simulink model "PowertrainModel"  (R2026b)
settings: Solver=VariableStepAuto
undefined symbols (not defined in the file): Powertrain
settings Model: DataDictionary=VehicleData.sldd  Creator=Xu Dingyi  LastModifiedBy=29358

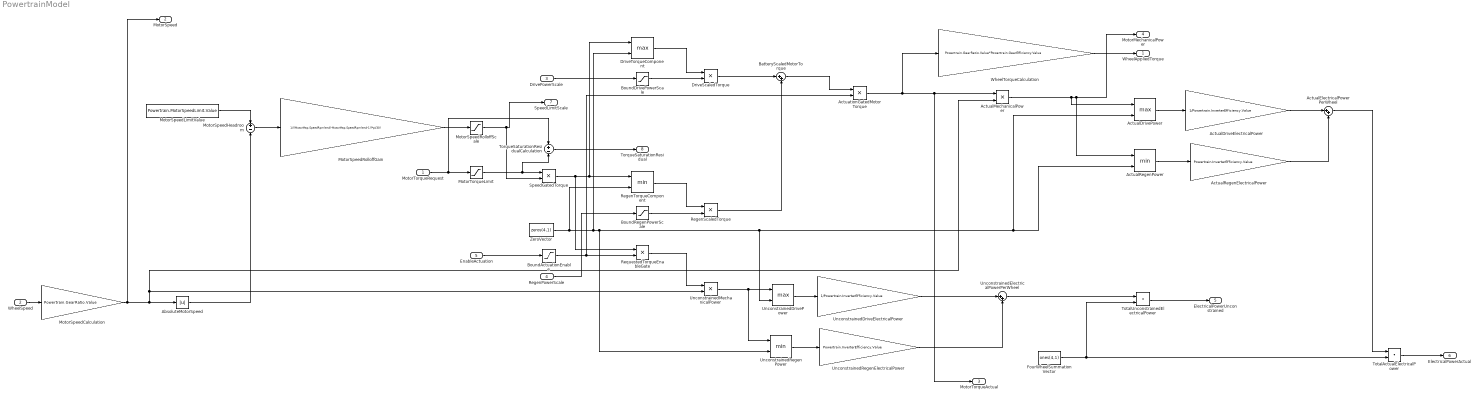
== system PowertrainModel ==
  MotorTorqueRequest : Inport  PortDimensions=[4 1]
  WheelSpeed : Inport  Port=2  PortDimensions=[4 1]
  DrivePowerScale : Inport  Port=3  PortDimensions=1
  RegenPowerScale : Inport  Port=4  PortDimensions=1
  EnableActuation : Inport  Port=5  PortDimensions=1
  AbsoluteMotorSpeed : Abs
  ActualDriveElectricalPower : Gain  Gain=1/Powertrain.InverterEfficiency.Value
  ActualDrivePower : MinMax  Function=max  Inputs=2
  ActualElectricalPowerPerWheel : Sum  Inputs=|++
  ActualMechanicalPower : Product  Inputs=**
  ActualRegenElectricalPower : Gain  Gain=Powertrain.InverterEfficiency.Value
  ActualRegenPower : MinMax  Inputs=2
  ActuationGatedMotorTorque : Product  Inputs=**
  BatteryScaledMotorTorque : Sum  Inputs=|++
  BoundActuationEnable : Saturate  UpperLimit=1  LowerLimit=0
  BoundDrivePowerScale : Saturate  UpperLimit=1  LowerLimit=0
  BoundRegenPowerScale : Saturate  UpperLimit=1  LowerLimit=0
  DriveScaledTorque : Product  Inputs=**
  DriveTorqueComponent : MinMax  Function=max  Inputs=2
  FourWheelSummationVector : Constant  Value=ones(4,1)
  MotorSpeedCalculation : Gain  Gain=Powertrain.GearRatio.Value
  MotorSpeedHeadroom : Sum  Inputs=+-
  MotorSpeedLimitValue : Constant  Value=Powertrain.MotorSpeedLimit.Value
  MotorSpeedRolloffGain : Gain  Gain=1/((MotorMap.SpeedRpm(end)-MotorMap.SpeedRpm(end-1))*pi/30)
  MotorSpeedRolloffScale : Saturate  UpperLimit=1  LowerLimit=0
  MotorTorqueLimit : Saturate  UpperLimit=Powertrain.MotorTorqueLimit.Value  LowerLimit=-Powertrain.MotorTorqueLimit.Value
  RegenScaledTorque : Product  Inputs=**
  RegenTorqueComponent : MinMax  Inputs=2
  RequestedTorqueEnableGate : Product  Inputs=**
  SpeedGatedTorque : Product  Inputs=**
  TorqueSaturationResidualCalculation : Sum  Inputs=+-
  TotalActualElectricalPower : DotProduct
  TotalUnconstrainedElectricalPower : DotProduct
  UnconstrainedDriveElectricalPower : Gain  Gain=1/Powertrain.InverterEfficiency.Value
  UnconstrainedDrivePower : MinMax  Function=max  Inputs=2
  UnconstrainedElectricalPowerPerWheel : Sum  Inputs=|++
  UnconstrainedMechanicalPower : Product  Inputs=**
  UnconstrainedRegenElectricalPower : Gain  Gain=Powertrain.InverterEfficiency.Value
  UnconstrainedRegenPower : MinMax  Inputs=2
  WheelTorqueCalculation : Gain  Gain=Powertrain.GearRatio.Value*Powertrain.GearEfficiency.Value
  ZeroVector : Constant  Value=zeros(4,1)
  WheelAppliedTorque : Outport
  MotorSpeed : Outport  Port=2
  MotorTorqueActual : Outport  Port=3
  MotorMechanicalPower : Outport  Port=4
  ElectricalPowerUnconstrained : Outport  Port=5
  ElectricalPowerActual : Outport  Port=6
  SpeedLimitScale : Outport  Port=7
  TorqueSaturationResidual : Outport  Port=8
  wires:
  ActualRegenPower/1 -> ActualRegenElectricalPower/1
  BoundActuationEnable/1 -> ActuationGatedMotorTorque/2, RequestedTorqueEnableGate/2
  MotorTorqueRequest/1 -> TorqueSaturationResidualCalculation/1, MotorTorqueLimit/1
  WheelSpeed/1 -> MotorSpeedCalculation/1
  TotalActualElectricalPower/1 -> ElectricalPowerActual/1
  RegenTorqueComponent/1 -> RegenScaledTorque/1
  MotorSpeedRolloffGain/1 -> MotorSpeedRolloffScale/1
  UnconstrainedRegenElectricalPower/1 -> UnconstrainedElectricalPowerPerWheel/2
  MotorSpeedLimitValue/1 -> MotorSpeedHeadroom/1
  TotalUnconstrainedElectricalPower/1 -> ElectricalPowerUnconstrained/1
  MotorSpeedCalculation/1 -> ActualMechanicalPower/2, UnconstrainedMechanicalPower/2, AbsoluteMotorSpeed/1, MotorSpeed/1
  ActuationGatedMotorTorque/1 -> MotorTorqueActual/1, ActualMechanicalPower/1, WheelTorqueCalculation/1
  MotorSpeedHeadroom/1 -> MotorSpeedRolloffGain/1
  AbsoluteMotorSpeed/1 -> MotorSpeedHeadroom/2
  RequestedTorqueEnableGate/1 -> UnconstrainedMechanicalPower/1
  MotorSpeedRolloffScale/1 -> SpeedLimitScale/1, SpeedGatedTorque/2
  UnconstrainedRegenPower/1 -> UnconstrainedRegenElectricalPower/1
  MotorTorqueLimit/1 -> TorqueSaturationResidualCalculation/2, SpeedGatedTorque/1
  EnableActuation/1 -> BoundActuationEnable/1
  DrivePowerScale/1 -> BoundDrivePowerScale/1
  TorqueSaturationResidualCalculation/1 -> TorqueSaturationResidual/1
  SpeedGatedTorque/1 -> DriveTorqueComponent/1, RegenTorqueComponent/1, RequestedTorqueEnableGate/1
  ZeroVector/1 -> ActualRegenPower/2, ActualDrivePower/2, UnconstrainedDrivePower/2, UnconstrainedRegenPower/2, DriveTorqueComponent/2, RegenTorqueComponent/2
  ActualElectricalPowerPerWheel/1 -> TotalActualElectricalPower/1
  BoundRegenPowerScale/1 -> RegenScaledTorque/2
  RegenPowerScale/1 -> BoundRegenPowerScale/1
  DriveTorqueComponent/1 -> DriveScaledTorque/1
  BoundDrivePowerScale/1 -> DriveScaledTorque/2
  DriveScaledTorque/1 -> BatteryScaledMotorTorque/1
  RegenScaledTorque/1 -> BatteryScaledMotorTorque/2
  UnconstrainedMechanicalPower/1 -> UnconstrainedRegenPower/1, UnconstrainedDrivePower/1
  BatteryScaledMotorTorque/1 -> ActuationGatedMotorTorque/1
  UnconstrainedDrivePower/1 -> UnconstrainedDriveElectricalPower/1
  UnconstrainedDriveElectricalPower/1 -> UnconstrainedElectricalPowerPerWheel/1
  WheelTorqueCalculation/1 -> WheelAppliedTorque/1
  ActualMechanicalPower/1 -> MotorMechanicalPower/1, ActualRegenPower/1, ActualDrivePower/1
  UnconstrainedElectricalPowerPerWheel/1 -> TotalUnconstrainedElectricalPower/1
  FourWheelSummationVector/1 -> TotalActualElectricalPower/2, TotalUnconstrainedElectricalPower/2
  ActualDrivePower/1 -> ActualDriveElectricalPower/1
  ActualDriveElectricalPower/1 -> ActualElectricalPowerPerWheel/1
  ActualRegenElectricalPower/1 -> ActualElectricalPowerPerWheel/2
